simulink model "sim_all"  (R2020a)
settings: Solver=VariableStepAuto  StartTime=0.0  StopTime=2000  RelTol=1e-3
values from neighbouring files (symbols this model uses):
  a1 = rho * D^4 * alpha1    (= 0.000388302366464)    [data_current.m]
  a2 = -rho * D^3 * alpha2 * (1 - omega)    (= 0.0037030698432)    [data_current.m]
  alpha1 = 0.0113    [data_current.m]
  alpha2 = -0.0091    [data_current.m]
  cornerA = [43.781381 ... (first row only)    [missionC.m]
  cornerB = [43.780975 ... (first row only)    [missionC.m]
  cornerC = [43.780189 ... (first row only)    [missionC.m]
  cornerD = [43.780602 ... (first row only)    [missionC.m]
  ctrl_clockwise = false    [controller.m]
  ctrl_int_bound_or = 0.1    [controller.m]
  ctrl_int_bound_pos = 1    [controller.m]
  ctrl_k_or = 1    [controller.m]
  ctrl_k_pos = 1/3    (= 0.333333333333)    [controller.m]
  ctrl_Ki_vel = 100    [controller.m]
  ctrl_Kp_v_pos = 200    [controller.m]
  ctrl_Kp_vel = 200    [controller.m]
  ctrl_TAM = [  1     1           0           0               0       0;               0     0           1           1               0       0;               0     0           0           0               1       1;               0     0  -(ctrl_r+ctrl_dc)  ctrl_r+ctrl_dc    0       0;               0     0           0           0            -ctrl_r    ctrl_r;           -ctrl_r ctrl_r        0           0       ...(+19 chars)    [controller.m]
  ctrl_Ts = 0.1    [controller.m]
  ctrl_va_uncontrolled = 0.15    [controller.m]
  ctrl_vel_uncontrolled = 0.5    [controller.m]
  D = 0.076    [data_current.m]
  dead_zone_limit = 31.5    [data_current.m]
  depth = 5    [missionC.m]
  distanceFromWall = 8    [missionC.m]
  initInspectedSide = 2    [missionC.m]
  initPoint = [ 43.780796 ... (first row only)    [missionC.m]
  mod_A = pi*mod_R*mod_R    [model.m]
  mod_Cd_F = 0.45    [model.m]
  mod_Cd_M = 0.4    [model.m]
  mod_eta_init = [mod_xNorth; mod_yEast; -mod_zDown; 0; 0; 0]    [model.m]
  mod_g = 9.81    [model.m]
  mod_h0 = 0    [model.m]
  mod_Ixx = mod_Io(1,1)    [model.m]
  mod_Iyy = mod_Io(2,2)    [model.m]
  mod_Izz = mod_Io(3,3)    [model.m]
  mod_Kp_dot = 0    [model.m]
  mod_lat0 = 43.780189    [model.m]
  mod_lon0 = 11.282698    [model.m]
  mod_m = 100    [model.m]
  mod_Mq_dot = mod_Kp_dot    (= 0)    [model.m]
  mod_ni_init = [0; 0; 0; 0; 0; 0]    [model.m]
  mod_Nr_dot = mod_Kp_dot    (= 0)    [model.m]
  mod_p1 = [0; mod_R; 0]    [model.m]
  mod_p2 = [0; -mod_R; 0]    [model.m]
  mod_p3 = [0; 0; (mod_R + mod_z_cm)]    [model.m]
  mod_p4 = [0; 0; -(mod_R + mod_z_cm)]    [model.m]
  mod_p5 = [mod_R; 0; 0]    [model.m]
  mod_p6 = [-mod_R; 0; 0]    [model.m]
  mod_R = ((3*mod_Vol)/(4*pi))^(1/3)    [model.m]
  mod_Rm = (4*mod_R)/(3*pi)    [model.m]
  mod_t1 = [1; 0; 0]    [model.m]
  mod_t2 = [1; 0; 0]    [model.m]
  mod_t3 = [0; 1; 0]    [model.m]
  mod_t4 = [0; 1; 0]    [model.m]
  mod_t5 = [0; 0; 1]    [model.m]
  mod_t6 = [0; 0; 1]    [model.m]
  mod_W = mod_m*mod_g    (= 981)    [model.m]
  mod_Xu_dot = (2/3)*mod_rho_AUV*pi*(mod_R^3)    [model.m]
  mod_Yv_dot = mod_Xu_dot    [model.m]
  mod_z_cm = mod_r_cm(3)    [model.m]
  mod_Zw_dot = mod_Xu_dot    [model.m]
  n_max = 340    [data_current.m]
  nav_DT = 0.1    [navigation.m]
  nav_filter = -1    [data_analysis_simulation_total.m]    (also in navigation.m)
  nav_giro = 2    [navigation.m]
  nav_h0 = 0    [navigation.m]
  nav_lat0 = cornerC(1)    [navigation.m]
  nav_lon0 = cornerC(2)    [navigation.m]
  nav_plane_AB = coefficient_plane(nav_A,nav_B)    [navigation.m]
  nav_plane_BC = coefficient_plane(nav_B,nav_C)    [navigation.m]
  nav_plane_CD = coefficient_plane(nav_C,nav_D)    [navigation.m]
  nav_plane_DA = coefficient_plane(nav_D,nav_A)    [navigation.m]
  nav_resampling = 10000    [navigation.m]
  omega = 0.1    [data_current.m]
  relativeDirection = 30    [missionC.m]
  res_enable_n_eff = 1    [navigation.m]
  rho = 1030    [data_current.m]
  sens_distCM = 0.267    [sensors.m]
  sens_Sample_time_AHRS = 0.1    [sensors.m]
  sens_Sample_time_depth = 0.1    [sensors.m]
  sens_Sample_time_dvl = 0.2    [sensors.m]
  sens_Sample_time_GPS = 1    [sensors.m]
  sens_Sample_time_GYRO = 0.1    [sensors.m]
  sens_Sample_time_sonar = 0.5    [sensors.m]
  sens_threshold = 0.485    [sensors.m]
  sens_Variance_AHRS_pitch = (0.0087)^2    (= 7.569e-05)    [sensors.m]
  sens_Variance_AHRS_roll = (0.0087)^2    (= 7.569e-05)    [sensors.m]
  sens_Variance_AHRS_yaw = (0.0017)^2    (= 2.89e-06)    [sensors.m]
  sens_Variance_depth1 = (0.2)^2    (= 0.04)    [sensors.m]
  sens_Variance_depth2 = (0.4)^2    (= 0.16)    [sensors.m]
  sens_Variance_DVL = (speed*0.03)^2    [sensors.m]
  sens_Variance_GPS = 3    [sensors.m]
  sens_Variance_GYRO = 2.5133e-06    [sensors.m]
  sens_Variance_sonar = 0.05    [sensors.m]
  soglia_or = [0.1, 0.1, 0.1]    [mission.m]
  soglia_orp = 0.1    [mission.m]
  soglia_parete = 0.5    [mission.m]
  soglia_parete_frenata = 0.5    [mission.m]
  soglia_pos = [0.00001, 0.00001, 0.5]    [mission.m]
  soglia_SOS_collisione = 2    [mission.m]
  soglia_SOS_or = [0.25, 0.25, 0.25]    [mission.m]
  soglia_SOS_orp = 0.25    [mission.m]
  soglia_SOS_parete = 1    [mission.m]
  soglia_SOS_pos = [0.00005, 0.00005, 1]    [mission.m]
  soglia_SOS_pos_ris = 2    [mission.m]
  soglia_SOS_vel = 0.2    [mission.m]
  SOS = 0    [mission.m]
  speed = 0.4    [missionC.m]
  stato = 100    [mission.m]
  timer = 40*2    (= 80)    [mission.m]
  Ts_supervisor = 0.1    [mission.m]
undefined symbols (not defined in the file or in its folder): DiscIntNeverNeededParam, nav_A, nav_B, nav_C, nav_D
libraries: simulink x8, cstblocks x6, simulink_extras x1
(part 5 of 8)

== matlab function sim_all/EKF/Calcolo distaza pareti/Calcolo orientazione dalla parete ==
  data: pos_es input; orient_parete output; parete_attuale input; orient input; nav_plane_AB parameter; nav_plane_BC parameter; nav_plane_CD parameter; nav_plane_DA parameter
function orient_parete  = orient_parete_calculator(pos_es, parete_attuale, orient, nav_plane_AB, nav_plane_BC, nav_plane_CD, nav_plane_DA)
    
    %consideriamo angoli di pitch e roll nulli, cioè si calcola
    %l'orientazione rispetto alla parete solo considerando rotazioni di yaw
    %(piano xy)

    Yaw   = orient(3);
    R_z = [cos(Yaw)     sin(Yaw)       0     ;
           -sin(Yaw)    cos(Yaw)       0     ;
              0            0           1    ];
    v_pos= R_z'*[1 0 0]';  %versore della retta lungo l'asse x (in body) in NED,
                       %cioè la direzione di riferimento di prua del veicolo     
    
    %selezione della parete di pattugliamento
switch parete_attuale                      
    case 1
        %% Piano di pattugliamento AB
        versore_plane_NED = [nav_plane_AB(1) nav_plane_AB(2) 0]';    %versore normale al piano
        versore_plane_NED = versore_plane_NED/norm(versore_plane_NED);

        %calcolo distanza e intersezione lungo la normale al piano
        t_ = -(pos_es(1)+nav_plane_AB(2)*pos_es(2)+nav_plane_AB(4))/(nav_plane_AB(2)*versore_plane_NED(2)+versore_plane_NED(1));
        inter_perp=zeros(3,1);
        inter_perp(1) = pos_es(1) + versore_plane_NED(1)*t_;
        inter_perp(2) = pos_es(2) + versore_plane_NED(2)*t_;
        inter_perp(3) = pos_es(3) + versore_plane_NED(3)*t_;
        
        %calcolo distanza e intersezione lungo la direzione di prua
        t_ = -(pos_es(1)+nav_plane_AB(2)*pos_es(2)+nav_plane_AB(4))/(nav_plane_AB(2)*v_pos(2)+v_pos(1));
        inter_prua=zeros(3,1);
        inter_prua(1) = pos_es(1) + v_pos(1)*t_;
        inter_prua(2) = pos_es(2) + v_pos(2)*t_;
        inter_prua(3) = pos_es(3) + v_pos(3)*t_;
        
        coef = nav_plane_AB;
        coef(4)=[];
        orient_parete = rad2deg(asin(abs(coef*v_pos)/(norm(coef)*norm(v_pos))));
        %se orient_parete è positiva, allora ci si trova tra - 90 e + 90 rispetto alla normale della parete 
        if t_ > 0              
            if inter_prua(1) > inter_perp(1) && inter_prua(2) < inter_perp(2)
                orient_parete = orient_parete - 90;
            else
                orient_parete = -(orient_parete - 90);
            end
        else
            if inter_prua(1) > inter_perp(1) && inter_prua(2) < inter_perp(2)
                orient_parete = (orient_parete + 90);
            else
                orient_parete = -(orient_parete + 90);
            end
        end    
    case 2
        %% Piano di pattugliamento BC
      	versore_plane_NED = [nav_plane_BC(1) nav_plane_BC(2) 0]';    %versore normale al piano
        versore_plane_NED = versore_plane_NED/norm(versore_plane_NED);

        %calcolo distanza e intersezione lungo la normale al piano
        t_ = -(pos_es(1)+nav_plane_BC(2)*pos_es(2)+nav_plane_BC(4))/(nav_plane_BC(2)*versore_plane_NED(2)+versore_plane_NED(1));
        inter_perp=zeros(3,1);
        inter_perp(1) = pos_es(1) + versore_plane_NED(1)*t_;
        inter_perp(2) = pos_es(2) + versore_plane_NED(2)*t_;
        inter_perp(3) = pos_es(3) + versore_plane_NED(3)*t_;

        %calcolo distanza e intersezione lungo la direzione di prua
        t_ = -(pos_es(1)+nav_plane_BC(2)*pos_es(2)+nav_plane_BC(4))/(nav_plane_BC(2)*v_pos(2)+v_pos(1));
        inter_prua=zeros(3,1);
        inter_prua(1) = pos_es(1) + v_pos(1)*t_;
        inter_prua(2) = pos_es(2) + v_pos(2)*t_;
        inter_prua(3) = pos_es(3) + v_pos(3)*t_;
        
        coef = nav_plane_BC;
        coef(4)=[];
        v_pos=-v_pos;
        orient_parete = rad2deg(asin(abs(coef*v_pos)/(norm(coef)*norm(v_pos))));
        %se orient_parete è positiva, allora ci si trova tra - 90 e + 90 rispetto alla normale della parete 
        if t_ > 0              
            if inter_prua(1) > inter_perp(1) && inter_prua(2) > inter_perp(2)
                orient_parete = orient_parete - 90;
            else
                orient_parete = -(orient_parete - 90);
            end
        else
            if inter_prua(1) > inter_perp(1) && inter_prua(2) > inter_perp(2)
                orient_parete = orient_parete + 90;
            else
                orient_parete = -(orient_parete + 90);
            end
        end
        
    case 3
        %% Piano di pattugliamento CD
      	versore_plane_NED = [nav_plane_CD(1) nav_plane_CD(2) 0]';    %versore normale al piano
        versore_plane_NED = versore_plane_NED/norm(versore_plane_NED);

        %calcolo distanza e intersezione lungo la normale al piano
        t_ = -(pos_es(1)+nav_plane_CD(2)*pos_es(2)+nav_plane_CD(4))/(nav_plane_CD(2)*versore_plane_NED(2)+versore_plane_NED(1));
        inter_perp=zeros(3,1);
        inter_perp(1) = pos_es(1) + versore_plane_NED(1)*t_;
        inter_perp(2) = pos_es(2) + versore_plane_NED(2)*t_;
        inter_perp(3) = pos_es(3) + versore_plane_NED(3)*t_;

        %calcolo distanza e intersezione lungo la direzione di prua
        t_ = -(pos_es(1)+nav_plane_CD(2)*pos_es(2)+nav_plane_CD(4))/(nav_plane_CD(2)*v_pos(2)+v_pos(1));
        inter_prua=zeros(3,1);
        inter_prua(1) = pos_es(1) + v_pos(1)*t_;
        inter_prua(2) = pos_es(2) + v_pos(2)*t_;
        inter_prua(3) = pos_es(3) + v_pos(3)*t_;
        
        coef = nav_plane_CD;
        coef(4)=[];
        v_pos=-v_pos;
        orient_parete = rad2deg(asin(abs(coef*v_pos)/(norm(coef)*norm(v_pos))));
        %se orient_parete è positiva, allora ci si trova tra - 90 e + 90 rispetto alla normale della parete 
        if t_ > 0              
            if inter_prua(1) > inter_perp(1) && inter_prua(2) < inter_perp(2)
                orient_parete = -orient_parete + 90;
            else
                orient_parete = orient_parete - 90;
            end
        else
             if inter_prua(1) > inter_perp(1) && inter_prua(2) < inter_perp(2)
                orient_parete = -orient_parete - 90;
            else
                orient_parete = orient_parete + 90;
            end
        end
        
    case 4
        %% Piano di pattugliamento DA
      	versore_plane_NED = [nav_plane_DA(1) nav_plane_DA(2) 0]';    %versore normale al piano
        versore_plane_NED = versore_plane_NED/norm(versore_plane_NED);

        %calcolo distanza e intersezione lungo la normale al piano
        t_ = -(pos_es(1)+nav_plane_DA(2)*pos_es(2)+nav_plane_DA(4))/(nav_plane_DA(2)*versore_plane_NED(2)+versore_plane_NED(1));
        inter_perp=zeros(3,1);
        inter_perp(1) = pos_es(1) + versore_plane_NED(1)*t_;
        inter_perp(2) = pos_es(2) + versore_plane_NED(2)*t_;
        inter_perp(3) = pos_es(3) + versore_plane_NED(3)*t_;

        %calcolo distanza e intersezione lungo la direzione di prua
        t_ = -(pos_es(1)+nav_plane_DA(2)*pos_es(2)+nav_plane_DA(4))/(nav_plane_DA(2)*v_pos(2)+v_pos(1));
        inter_prua=zeros(3,1);
        inter_prua(1) = pos_es(1) + v_pos(1)*t_;
        inter_prua(2) = pos_es(2) + v_pos(2)*t_;
        inter_prua(3) = pos_es(3) + v_pos(3)*t_;
        
        coef = nav_plane_DA;
        coef(4)=[];
        orient_parete = rad2deg(asin(abs(coef*v_pos)/(norm(coef)*norm(v_pos))));
        %se orient_parete è positiva, allora ci si trova tra - 90 e + 90 rispetto alla normale della parete 
        if t_ > 0              
            if inter_prua(1) < inter_perp(1) && inter_prua(2) < inter_perp(2)
                orient_parete = orient_parete - 90;
            else
                orient_parete = -orient_parete + 90;
            end
        else
            if inter_prua(1) < inter_perp(1) && inter_prua(2) < inter_perp(2)
                orient_parete = orient_parete + 90;
            else
                orient_parete = -orient_parete - 90;
            end
        end
        
    otherwise
        %%
       coef=[0 0 0 0];
       orient_parete = NaN;
end
    
    
end

== matlab function sim_all/EKF/ECEF2NED ==
  data: GPS_ECEF input; GPS_NED output; nav_lat0 parameter; nav_lon0 parameter; nav_h0 parameter
%Componente di ingresso in terna ECEF
%Lat  [gradi]
%Long  [gradi]
%flag data_valid

function GPS_NED = GPS_conv_valid(GPS_ECEF, nav_lat0, nav_lon0, nav_h0)
    
    coder.extrinsic('evalin', 'wgs84Ellipsoid', 'geodetic2ned');

    if GPS_ECEF(3)==1
        GPS_NED = zeros(3,1);
        [GPS_NED(1),GPS_NED(2),GPS_NED(3)]= geodetic2ned(GPS_ECEF(1),GPS_ECEF(2),0,nav_lat0,nav_lon0,nav_h0,wgs84Ellipsoid);
        GPS_NED(3) = GPS_ECEF(3);
    else                            %qui non si effettua la conversione se il dato non è valido
        GPS_NED = GPS_ECEF; 
    end
end

== matlab function sim_all/EKF/Extended Kalman Filter/AHRS__check/MATLAB Function4 ==
  data: flag_AHRS output; AHRS_new input; AHRS_now output; AHRS_old input
%gestione di misura errata di AHRS
function [flag_AHRS, AHRS_now] = fcn(AHRS_new, AHRS_old)

    if isnan(AHRS_new(1,1)) || isnan(AHRS_new(2,1)) || isnan(AHRS_new(3,1))
        AHRS_now = AHRS_old;
        flag_AHRS = 1;
        disp('Misura AHRS non valida')
    else
        AHRS_now = AHRS_new;
        flag_AHRS = 0;
    end  
end

== matlab function sim_all/EKF/Extended Kalman Filter/CORREZIONE/MATLAB Function ==
  data: x_k_k_1 input; x_k output; P_k_k_1 input; e input size=6 1; H input size=6 3; R_k input size=6 6; P_k output; nav_flag_init input
%%Passo di Correzione

function [x_k, P_k] = correction(x_k_k_1,P_k_k_1, e, H, R_k,nav_flag_init)
    
     x_k = zeros(3,1);
     P_k = zeros(3,3);
     
     
    if nav_flag_init ~= 0
        %matrice ottenuta da derivata di funzione h (6x1) per i rumori sei vari
        %sensori, che sono 6. (ha dimensione 6x6)
        %andrebbero anche considerati i rumori legati all'AHRS che al momento
        %sono trascurati
        %M = eye(6,6);              %M è l'dientità
        S_k = H*P_k_k_1*H'+ R_k;
        K_k = P_k_k_1*H'*(inv(S_k));

        P_k = (eye(3)-(K_k*H))*P_k_k_1;
        x_k = x_k_k_1 + K_k * e;
    end

end

== matlab function sim_all/Mission_supervisor_v3/Mission_Supervisor/Immersione/MATLAB Function ==
  data: soglia_pos parameter; delta_current_immers output; delta_stato_immers output; Pos_d output size=3; Or_d output size=3; Pos_s input; depth parameter; punto_iniz_patt input; Or_in input; error_flag input; soglia_SOS_pos parameter; SOS parameter
function [delta_current_immers, delta_stato_immers, Pos_d, Or_d]=Immersione(soglia_pos, Pos_s, depth, punto_iniz_patt, Or_in, error_flag, soglia_SOS_pos, SOS)

    disp("Immersione");
    
    %% Unità di misura 
    
    % Pos_d, Pos_s, punto_iniz_patt, soglia_pos, soglia_SOS_pos            [deg, deg, m]
    % Or_d, Or_in                                                          [rad, rad, rad]
    % distanceFromWall, depth                                              [m]


    %% Inizializzazione variabili
    
    % Utilizzata durante la permanenza nello stato corrente
    delta_stato_immers = 0;
    
    pronti = false; 
    
    %% Preparazione dei riferimenti da fornire ai blocchi successivi
    
    % Posizione da raggiungere
    Pos_d = [punto_iniz_patt(1); punto_iniz_patt(2); depth];
                                                                            %*****TEST******%
                                                                            %Pos_d = [43; 11; 0];
    
    % Orientazione da mantenere
    Or_d = Or_in;
    
    % Transizione di stato effettiva
    delta_current_immers = 103 - 102;  
        
       
    %% Verifiche
    
    % Verifica della corretta posizione
    if (abs(Pos_s(1) - Pos_d(1)) > soglia_SOS_pos(1) || ...
        abs(Pos_s(2) - Pos_d(2)) > soglia_SOS_pos(2))
    
        SOS = 1;
        disp("EMERGENZA:"); 
        
        if (abs(Pos_s(1) - Pos_d(1)) > soglia_SOS_pos(1))
            disp("Rilevato errore sulla posizione X");
        end
        
        if (abs(Pos_s(2) - Pos_d(2)) > soglia_SOS_pos(2))
            disp("Rilevato errore sulla posizione Y");
        end

    end
    
    if error_flag == 1
        disp("EMERGENZA: errore segnalato dagli altri sottosistemi");
        SOS = 1;
    end
    
    % Si verifica di aver raggiunto la profondità desiderata 
    if (SOS == 0 && ...
        abs(Pos_s(3) - Pos_d(3)) < soglia_pos(3))
    
        pronti = true;
    end
    
    
    %% Decisione dello stato successivo
    
    if pronti == true
        
        delta_stato_immers = 104 - 103; % Transizione eseguita correttamente
    end 
    if SOS == 1
            
            delta_stato_immers = 301 - 103; % Transizione nello stato di emergenza
    end
    % Si rimane nello stato corrente

end

== matlab function sim_all/EKF/Extended Kalman Filter/Creazione vettore delle misure ==
  data: flag_vect output; GPS input; mis_vect output; depth input; s_pr input; s_dx input; s_sx input; mis_vect_prec input; J input; pos input; nav_plane_AB parameter; nav_plane_BC parameter; nav_plane_CD parameter; nav_plane_DA parameter; nav_A parameter; nav_B parameter; nav_C parameter; nav_D parameter; distanceFromWall parameter; flag_DVL input; flag_AHRS input
%%
% Questa funzione impila le informazioni derivanti dai vari sensori in un
% unico vettore mis_vect 7x1.                                 
% Ci sarà un corrispondente vettore flag_vect 7x1 di flag che sarà pari a:

% flag(i) = 0  se la misura è uguale a quella arrivata nell'istante
% predecente, in tal caso la correzione non verrà effettuata
% flag(i) = 1 se la misura è stata aggiornata rispetto a quella precendente
 
% NB il controllo sulla validità dei dati del GPS è valutata nel blocco
% sucessivo

function [flag_vect,mis_vect] = misure_vector(GPS,depth,s_pr,s_dx,s_sx, mis_vect_prec,...
          J, pos, nav_plane_AB, nav_plane_BC, nav_plane_CD, nav_plane_DA, nav_A, nav_B, nav_C, nav_D, distanceFromWall, ...
          flag_DVL, flag_AHRS)
    
    mis_vect = zeros(7,1);
    flag_vect = zeros(7,1);
	mis_vect = [GPS(1) GPS(2) GPS(3) depth s_pr s_dx s_sx]';
    
    for i=[1:7]
        if mis_vect(i) ~= mis_vect_prec(i)
            flag_vect(i) = 1;
        end
    end
    
    %si valuta se la misura del profondimetro è valida
    if isnan(depth)  
        flag_vect(4) = 0;
    end
     
    %si controlla che sia disponibile il dato dai sonar
    if isnan(s_pr)
        flag_vect(5) = 0;
    end
    if isnan(s_dx)
        flag_vect(6) = 0;
    end
    if isnan(s_sx)
        flag_vect(7) = 0;
    end
    
    %se i dati dei sonar qui sono utilizzabili, è necessario assicurarci che il 
    %loro raggio non punti verso uno spigolo, in quel caso potrebbe
    %causare una correzione errata
    if flag_vect(5) == 1               %se i dati del sonar di prua sono nuovi
            versore_son_NED = J*[1 0 0]';          %versore terna NED sonar prua
            flag_vect(5) = inter(pos, versore_son_NED ,nav_plane_AB,nav_plane_BC,nav_plane_CD,nav_plane_DA, nav_A, nav_B, nav_C, nav_D);       
    end

        if flag_vect(6) == 1               %se i dati del sonar destro sono nuovi
                versore_son_NED = J*[0 1 0]';          %versore terna NED sonar dx
                flag_vect(6) = inter(pos, versore_son_NED ,nav_plane_AB,nav_plane_BC,nav_plane_CD,nav_plane_DA, nav_A, nav_B, nav_C, nav_D);       
        end
        if flag_vect(7) == 1               %se i dati del sonar sinistro sono nuovi
                versore_son_NED = J*[0 -1 0]';          %versore terna NED sonar sx
                flag_vect(7) = inter(pos, versore_son_NED ,nav_plane_AB,nav_plane_BC,nav_plane_CD,nav_plane_DA, nav_A, nav_B, nav_C, nav_D);
        end 
%         la terza componente di flag_vect non sarà utilizzata. per assicurarci
%         che i dati del GPS siano validi ci rifaremo sempre su mis_vect


    if flag_DVL == 0 && flag_AHRS == 0  %i sonar vengono usati sempre nella correzione se un sensore tra DLV
                                        %o AHRS non funziona momentaneamente 
        
        soglia_distanza=distanceFromWall*3;
        soglia_variazione=0.8;
        if  mis_vect(5) > soglia_distanza || abs(mis_vect(5)- mis_vect_prec(5)) > soglia_variazione
            flag_vect(5) = 0;
        end
        if  mis_vect(6) > soglia_distanza || abs(mis_vect(6)- mis_vect_prec(6)) > soglia_variazione
            flag_vect(6) = 0;
        end
        if  mis_vect(7) > soglia_distanza || abs(mis_vect(7)- mis_vect_prec(7)) > soglia_variazione
            flag_vect(7) = 0;
        end
    end
end




function [flag] = inter(pos, versore_son_NED,nav_plane_AB,nav_plane_BC,nav_plane_CD,nav_plane_DA, nav_A, nav_B, nav_C, nav_D)
    
    %calcolo della distanza dalla posizione ai piani delle pareti seguendo
    %la direzione data dal versore del sonar

    t_AB = -(pos(1)+nav_plane_AB(2)*pos(2)+nav_plane_AB(4))/(nav_plane_AB(2)*versore_son_NED(2)+versore_son_NED(1));
    t_BC = -(pos(1)+nav_plane_BC(2)*pos(2)+nav_plane_BC(4))/(nav_plane_BC(2)*versore_son_NED(2)+versore_son_NED(1));
    t_CD = -(pos(1)+nav_plane_CD(2)*pos(2)+nav_plane_CD(4))/(nav_plane_CD(2)*versore_son_NED(2)+versore_son_NED(1));
    t_DA = -(pos(1)+nav_plane_DA(2)*pos(2)+nav_plane_DA(4))/(nav_plane_DA(2)*versore_son_NED(2)+versore_son_NED(1));
    
    if t_AB < 0
        t_AB = inf;
    end
    if t_BC < 0
        t_BC = inf;
    end
    if t_CD < 0
        t_CD = inf;
    end
    if t_DA < 0
        t_DA = inf;
    end
           
    [dist, index] = min([t_AB t_BC t_CD t_DA]);
    dist = dist - 0.267;       %va tolto il raggio del veicolo rispetto al centro di massa
    
    int=zeros(1,3);
    %calcolo l'intersezione
    int(1) = pos(1) + versore_son_NED(1)*dist;
    int(2) = pos(2) + versore_son_NED(2)*dist;
    int(3) = 0;
    
    soglia_spigolo = 5;          %distanza massima dallo spigolo entro la quale 
                       %la misura del sonar non è buona
    flag=1;
    switch index
        case 1      
            if norm(int-nav_A) < soglia_spigolo || norm(int-nav_B) < soglia_spigolo
                flag=0;
            end
        case 2
            if norm(int-nav_B) < soglia_spigolo || norm(int-nav_C) < soglia_spigolo
                flag=0;
            end
        case 3
            if norm(int-nav_C) < soglia_spigolo || norm(int-nav_D) < soglia_spigolo
                flag=0;
            end
        case 4
            if norm(int-nav_D) < soglia_spigolo || norm(int-nav_A) < soglia_spigolo
                flag=0;
            end
        otherwise
            disp('errore nella intersezione del piano')
    end
end

== matlab function sim_all/EKF/Extended Kalman Filter/DVL_check/MATLAB Function4 ==
  data: flag_DVL output; DVL_new input; DVL_now output; DVL_old input
%gestione di misura errata del DVL
function [flag_DVL, DVL_now] = fcn(DVL_new, DVL_old)

    if isnan(DVL_new(1,1)) || isnan(DVL_new(2,1)) || isnan(DVL_new(3,1))
        DVL_now = DVL_old;
        flag_DVL = 1;
        disp('Misura DVL non valida')
    else
        DVL_now = DVL_new;
        flag_DVL = 0;
    end  
end

== matlab function sim_all/EKF/Extended Kalman Filter/MATLAB Function ==
  data: GPS input; x0 output; depth input; P0 output; flag input; flag output
%blocco di inizializzazione del Filtro

function [x0, P0, flag] = EKF_init(GPS, depth, flag)
    
    x0 = zeros(3,1);
    P0 = zeros(3,3);
    
    % il valore di nav_flag_init è all'inizio della simulazione pari a 0
    % appena c'è il primo dato disponibile del GPS (insieme al profondimetro)
    % si assume quella come punto di inizializzazione del filtro.

    if flag == 0
        if GPS(3)==1
            x0 = [GPS(1), GPS(2), depth]';
            P0 = diag([3 3 (0.2)^2]);       %sono le varianze del GPS e del profondimetro (come nella R)
            flag = 1;                   %se vale 1 bisogna assegnare i primi valori a x_k_1 e P_k_1
        end
               
    end

end

== matlab function sim_all/EKF/Extended Kalman Filter/MATLAB Function1 ==
  data: orient input; J output
%calcolo matrice J
function J = calcolo_jacobiano(orient)

    Roll  = orient(1);
    Pitch = orient(2);
    Yaw   = orient(3);

    R_x = [ 1               0              0;
            0           cos(Roll)     sin(Roll);
            0           -sin(Roll)    cos(Roll)];

    R_y = [cos(Pitch)       0   -sin(Pitch);
              0             1         0;
           sin(Pitch)       0   cos(Pitch)];

    R_z = [cos(Yaw)     sin(Yaw)      0;
          -sin(Yaw)     cos(Yaw)      0;
              0            0          1];

    J = (R_z'*R_y')*R_x';
end

== matlab function sim_all/EKF/Extended Kalman Filter/MATLAB Function2 ==
  data: u_k_1 input; orient input; L output
%calcolo matrice L
function L = calcolo_L(u_k_1,orient)

    L =  [   u_k_1(2)*((sin(orient(1))*sin(orient(3)))/10 + (cos(orient(1))*cos(orient(3))*sin(orient(2)))/10) + u_k_1(3)*((cos(orient(1))*sin(orient(3)))/10 - (cos(orient(3))*sin(orient(1))*sin(orient(2)))/10), (u_k_1(3)*cos(orient(1))*cos(orient(3))*cos(orient(2)))/10 - (u_k_1(1)*cos(orient(3))*sin(orient(2)))/10 + (u_k_1(2)*cos(orient(3))*cos(orient(2))*sin(orient(1)))/10, u_k_1(3)*((cos(orient(3))*sin(orient(1)))/10 - (cos(orient(1))*sin(orient(3))*sin(orient(2)))/10) - u_k_1(2)*((cos(orient(1))*cos(orient(3)))/10 + (sin(orient(1))*sin(orient(3))*sin(orient(2)))/10) - (u_k_1(1)*cos(orient(2))*sin(orient(3)))/10, (cos(orient(3))*cos(orient(2)))/10, (cos(orient(3))*sin(orient(1))*sin(orient(2)))/10 - (cos(orient(1))*sin(orient(3)))/10, (sin(orient(1))*sin(orient(3)))/10 + (cos(orient(1))*cos(orient(3))*sin(orient(2)))/10;...
           - u_k_1(2)*((cos(orient(3))*sin(orient(1)))/10 - (cos(orient(1))*sin(orient(3))*sin(orient(2)))/10) - u_k_1(3)*((cos(orient(1))*cos(orient(3)))/10 + (sin(orient(1))*sin(orient(3))*sin(orient(2)))/10), (u_k_1(3)*cos(orient(1))*cos(orient(2))*sin(orient(3)))/10 - (u_k_1(1)*sin(orient(3))*sin(orient(2)))/10 + (u_k_1(2)*cos(orient(2))*sin(orient(1))*sin(orient(3)))/10, u_k_1(3)*((sin(orient(1))*sin(orient(3)))/10 + (cos(orient(1))*cos(orient(3))*sin(orient(2)))/10) - u_k_1(2)*((cos(orient(1))*sin(orient(3)))/10 - (cos(orient(3))*sin(orient(1))*sin(orient(2)))/10) + (u_k_1(1)*cos(orient(3))*cos(orient(2)))/10, (cos(orient(2))*sin(orient(3)))/10, (cos(orient(1))*cos(orient(3)))/10 + (sin(orient(1))*sin(orient(3))*sin(orient(2)))/10, (cos(orient(1))*sin(orient(3))*sin(orient(2)))/10 - (cos(orient(3))*sin(orient(1)))/10;...
                                                                                                             (u_k_1(2)*cos(orient(1))*cos(orient(2)))/10 - (u_k_1(3)*cos(orient(2))*sin(orient(1)))/10,                                      - (u_k_1(1)*cos(orient(2)))/10 - (u_k_1(3)*cos(orient(1))*sin(orient(2)))/10 - (u_k_1(2)*sin(orient(1))*sin(orient(2)))/10,                                                                                                                                                                                                                              0,               -sin(orient(2))/10,                                               (cos(orient(2))*sin(orient(1)))/10,                                               (cos(orient(1))*cos(orient(2)))/10]; 
end

== matlab function sim_all/EKF/Extended Kalman Filter/MATLAB Function3 ==
  data: flag_vect input; mis_vect input; R_ input size=6 6; R_k output size=6 6
%calcolo matrice R
function R_k = R_cutter(flag_vect, mis_vect,R_)
%valutazione misure GPS
    R=R_;   
    i=0;
    if mis_vect(3) == 0                    %se i dati del GPS non sono validi
        R(1,:) = [];
        R(:,1) = [];
        i=i+1;
        R(2-i,:) = [];
        R(:,2-i) = [];
        i=i+1;
        if flag_vect(4) == 0               %se i dati del profondimetro non sono nuovi
            R(3-i,:) = [];
            R(:,3-i) = [];
            i=i+1;
        end
        if flag_vect(5) == 0               %se i dati del sonar di prua non sono nuovi
            R(4-i,:) = [];
             R(:,4-i) = [];
            i=i+1;
        end
        if flag_vect(6) == 0               %se i dati del sonar sinistro non sono nuovi
            R(5-i,:) = [];
             R(:,5-i) = [];
            i=i+1;
        end
        if flag_vect(7) == 0               %se i dati del sonar destro non sono nuovi
            R(6-i,:) = [];
             R(:,6-i) = [];
        end
    % da qui invece abbiamo il GPS valido
    else
        if flag_vect(1)==0 || flag_vect(2)==0  %se i dati del GPS non sono nuovi
            R(1-i,:) = [];
            R(:,1-i) = [];
            i=i+1;
            R(2-i,:) = [];
            R(:,2-i) = [];
            i=i+1;
        end
       
        if flag_vect(4) == 0               %se i dati del profondimetro non sono nuovi
            R(3-i,:) = [];
            R(:,3-i) = [];
            i=i+1;
        end
       
        R(4-i,:) = []; %annulliamo le misure dei sonar
        R(:,4-i) = [];         
        i=i+1;
        R(5-i,:) = [];
        R(:,5-i) = [];
        i=i+1;
        R(6-i,:) = [];
        R(:,6-i) = [];
       
    end
    R_k=R;
end

== matlab function sim_all/EKF/Extended Kalman Filter/MISURA VIRTUALE/MATLAB Function ==
  data: x_k_k_1 input; flag_vect input; mis_vect input; e output size=6 1; H output size=6 3; J input; nav_plane_AB parameter; nav_plane_BC parameter; nav_plane_CD parameter; nav_plane_DA parameter
%calcolo  misure virtuali
function [e, H] = virtual(x_k_k_1, flag_vect, mis_vect, J, nav_plane_AB, nav_plane_BC, nav_plane_CD, nav_plane_DA)

    e = zeros(6,1);
    h = zeros(6,1);
    z = zeros(6,1);
    H = zeros(6,3);
    
    
    %valutazione misure GPS
    if mis_vect(3)==1                                   %se i dati del GPS sono validi
        if flag_vect(1) == 1 && flag_vect(2) == 1       %se i dati del GPS sono nuovi
            
            z = z + [mis_vect(1) mis_vect(2) 0 0 0 0]';
            h = h + [x_k_k_1(1)   x_k_k_1(2) 0 0 0 0]';
        
            H(1,:)= [1 0 0];
            H(2,:)= [0 1 0];
        end
    end
    
    %valutazione misure depth
    if flag_vect(4) == 1                                 %se i dati del profondimetro sono nuovi
            
        z = z + [0 0 mis_vect(4) 0 0 0]'; 
        h = h + [0 0  x_k_k_1(3) 0 0 0]';

        H(3,:)= [0 0 1];
    end
    
    %valutiamo ora le misure virtuali solo se quelle del GPS non sono
    %valide
    if mis_vect(3)==0                      %se i dati del GPS non sono validi
        
        if flag_vect(5) == 1               %se i dati del sonar di prua sono nuovi
                
                versore_son_NED = J*[1 0 0]';          %versore terna NED sonar prua
                
                [distanza, plane] = inter(x_k_k_1, versore_son_NED ,nav_plane_AB,nav_plane_BC,nav_plane_CD,nav_plane_DA);
                z = z + [0 0 0 mis_vect(5) 0 0]'; 
                h = h + [0 0 0 distanza    0 0]';
                
                H_new=zeros(1,3);
                [H_new(1), H_new(2), H_new(3)] = calc_H_vect(x_k_k_1, versore_son_NED,plane);
                H(4,:) = H_new;                
        end
    
        if flag_vect(6) == 1               %se i dati del sonar destro sono nuovi
                
                versore_son_NED = J*[0 1 0]';          %versore terna NED sonar dx
                
                [distanza, plane] = inter(x_k_k_1, versore_son_NED ,nav_plane_AB,nav_plane_BC,nav_plane_CD,nav_plane_DA);
                z = z + [0 0 0 0 mis_vect(6) 0]'; 
                h = h + [0 0 0 0 distanza    0]';
                
                H_new=zeros(1,3);
                [H_new(1), H_new(2), H_new(3)] = calc_H_vect(x_k_k_1, versore_son_NED,plane);
                H(5,:) = H_new;
        end
    
        if flag_vect(7) == 1               %se i dati del sonar sinistro sono nuovi
                 
                versore_son_NED = J*[0 -1 0]';          %versore terna NED sonar sx
                
                [distanza, plane] = inter(x_k_k_1, versore_son_NED ,nav_plane_AB,nav_plane_BC,nav_plane_CD,nav_plane_DA);
                z = z + [0 0 0 0 0 mis_vect(7)]'; 
                h = h + [0 0 0 0 0 distanza   ]'; 
                
                H_new=zeros(1,3);
                [H_new(1), H_new(2), H_new(3)] = calc_H_vect(x_k_k_1, versore_son_NED,plane);
                H(6,:) = H_new;
        end
    end
    
    e = z - h;
    
    %%si riducono le dimensioni della matrice H e del vettore e
    
    i=0;
    if mis_vect(3) == 0                    %se i dati del GPS non sono validi
        H(1-i,:) = [];
        e(1-i) = [];
        i=i+1;
        H(2-i,:) = [];
        e(2-i) = [];
        i=i+1;
        if flag_vect(4) == 0               %se i dati del profondimetro non sono nuovi
            H(3-i,:) = [];
            e(3-i) = [];
            i=i+1;
        end
        if flag_vect(5) == 0               %se i dati del sonar di prua non sono nuovi
            H(4-i,:) = [];
            e(4-i) = [];
            i=i+1;
        end
        if flag_vect(6) == 0               %se i dati del sonar sinistro non sono nuovi
            H(5-i,:) = [];
            e(5-i) = [];
            i=i+1;
        end
        if flag_vect(7) == 0               %se i dati del sonar destro non sono nuovi
            H(6-i,:) = [];
            e(6-i) = [];
        end
    % da qui invece si ha il GPS valido
    else
        if flag_vect(1)==0 || flag_vect(2)==0  %se i dati del GPS non sono nuovi
            H(1-i,:) = [];
            e(1-i) = [];
            i=i+1;
            H(2-i,:) = [];
            e(2-i) = [];
            i=i+1;
        end
        
        if flag_vect(4) == 0               %se i dati del profondimetro non sono nuovi
            H(3-i,:) = [];
            e(3-i) = [];
            i=i+1;
        end
        
        H(4-i,:) = [];                      %annulliamo le misure dei sonar
        e(4-i) = [];
        i=i+1;
        H(5-i,:) = [];
        e(5-i) = [];
        i=i+1;
        H(6-i,:) = [];        
        e(6-i) = [];    
    end
    i=0;
end



%%
%%%%%%%%%%%%%%%%%%%%%%%%%%%%%%%%%%%%%%%%%%%%%%%%%%%%%%%%%%%%%%%%%%%%%%%%%%%%%%%%%%%%%%%%

function [dist, plane] = inter(pos, versore_son_NED,nav_plane_AB,nav_plane_BC,nav_plane_CD,nav_plane_DA)
    
    %calcolo della distanza dalla posizione ai piani delle pareti seguendo
    %la direzione data dal versore del sonar

    t_AB = -(pos(1)+nav_plane_AB(2)*pos(2)+nav_plane_AB(4))/(nav_plane_AB(2)*versore_son_NED(2)+versore_son_NED(1));
    t_BC = -(pos(1)+nav_plane_BC(2)*pos(2)+nav_plane_BC(4))/(nav_plane_BC(2)*versore_son_NED(2)+versore_son_NED(1));
    t_CD = -(pos(1)+nav_plane_CD(2)*pos(2)+nav_plane_CD(4))/(nav_plane_CD(2)*versore_son_NED(2)+versore_son_NED(1));
    t_DA = -(pos(1)+nav_plane_DA(2)*pos(2)+nav_plane_DA(4))/(nav_plane_DA(2)*versore_son_NED(2)+versore_son_NED(1));
    
    if t_AB < 0
        t_AB = inf;
    end
    if t_BC < 0
        t_BC = inf;
    end
    if t_CD < 0
        t_CD = inf;
    end
    if t_DA < 0
        t_DA = inf;
    end
           
    [dist, index] = min([t_AB t_BC t_CD t_DA]);
    dist = dist - 0.267;       %va tolto il raggio del robot rispetto al centro di massa
    
    switch index
        case 1
            plane = nav_plane_AB;
        case 2
            plane = nav_plane_BC;
        case 3
            plane = nav_plane_CD;
        case 4
            plane = nav_plane_DA;
        otherwise
            plane=[0 0 0 0];
            disp('errore nella intersezione del piano')
    end
    
end

function [H1, H2, H3]= calc_H_vect(pos, sonar, plane)

    H1 = sign(pos(1) + plane(4) + pos(2)*plane(2))/abs(sonar(1) + plane(2)*sonar(2));
    H2 = (plane(2)*sign(pos(1) + plane(4) + pos(2)*plane(2)))/abs(sonar(1) + plane(2)*sonar(2));   
    H3 = 0;
end

== matlab function sim_all/EKF/Extended Kalman Filter/PREDIZIONE/Passo di Predizione ==
  data: x0 input; P0 input; x_k_1 input; u_k_1 input; x_k output; P_k_1 input; P_k output size=3 3; J input; L input; Q_k_1 input; nav_DT parameter; nav_flag_init input; nav_flag_init output
%% Passo di PREDIZIONE

function [x_k,  P_k, nav_flag_init] = prediction(x0, P0, x_k_1, u_k_1,  P_k_1, J, L, Q_k_1, nav_DT, nav_flag_init)
    
    x_k = zeros(3,1);
    P_k = zeros(3,3);

    % il valore di nav_flag_init all'inizio della simulazione é pari a 0
    % appena c'è il primo dato disponibile del GPS (insieme al profondimetro)
    % si assume quella come punto di inizializzazione del filtro.

    if nav_flag_init ~= 0      
        if nav_flag_init == 1
            x_k_1 = x0;
            P_k_1 = P0;
            nav_flag_init = 2;      % =2 così l'inizializzazione è fatta una sola volta.
        end
        
        %passo di predizione       
        x_k = x_k_1 + nav_DT*J*u_k_1;
        P_k = P_k_1 + L*Q_k_1*L';               %la matrice F è F = I
           
    end
end

== matlab function sim_all/EKF/Extended Kalman Filter/Q_error/MATLAB Function4 ==
  data: Q input; Q_k_1 input; Q_k output; flag_AHRS input; flag_DVL input
%calcolo matrice Q
function Q_k = fcn(Q, Q_k_1, flag_AHRS, flag_DVL)

    Q_k = Q;
    
    K=10;
    if flag_DVL == 1
       Q_k = Q_k_1 + K*5*diag([0,0,0,(0.012)^2,(0.012)^2,(0.012)^2]);
    end
    
    if flag_AHRS == 1
       Q_k = Q_k_1 + K*50*diag([(0.0087)^2, (0.0087)^2, (0.0017)^2,0,0,0]);  
    end
        
end

== matlab function sim_all/EKF/Gyro_check/MATLAB Function4 ==
  data: flag_gyro output; gyro_new input; gyro_now output; gyro_old input
% gestione di misura errata del giroscopio
function [flag_gyro, gyro_now] = fcn(gyro_new, gyro_old)

    if isnan(gyro_new(1,1)) || isnan(gyro_new(2,1)) || isnan(gyro_new(3,1))
        gyro_now = gyro_old;
        flag_gyro = 1;
        disp('Misura gyro non valida')
    else
        gyro_now = gyro_new;
        flag_gyro = 0;
    end  
end

== matlab function sim_all/EKF/MATLAB Function ==
  data: u input; y output
function y = Wrap2pi(u)
y = [0;0;0];
coder.extrinsic('wrapToPi');
y = wrapToPi(u);
end

== matlab function sim_all/EKF/NED2ECEF ==
  data: pos_es_NED input; pos_es_ECEF output; nav_lat0 parameter; nav_lon0 parameter; nav_h0 parameter
%%Blocco di conversione NED2ECEF

function pos_es_ECEF = pos_NED2ECEF(pos_es_NED,nav_lat0, nav_lon0, nav_h0)
     
    coder.extrinsic('evalin', 'wgs84Ellipsoid', 'ned2geodetic');
    pos_es_ECEF = zeros(3,1);
    depth = pos_es_NED(3); 
    
    [pos_es_ECEF(1),pos_es_ECEF(2),pos_es_ECEF(3)]= ned2geodetic(pos_es_NED(1),pos_es_NED(2),0,nav_lat0,nav_lon0,nav_h0,wgs84Ellipsoid);
    pos_es_ECEF(3) = depth;
end

== matlab function sim_all/EKF/SOS_flag_generator/MATLAB Function ==
  data: P_es input; SOS output; DVL input; AHRS input; gyro input; contatore input size=3 1; contatore output
%% Generazione flag di emergenza
% 1. Assenza di segnali dai sensori per un determinato tempo

function [SOS, contatore] = SOS_flag(P_es, DVL, AHRS, gyro, contatore)
    SOS=0;
 
    soglia_P = 10; %[m^2]
    if P_es(1,1)+P_es(2,2) > soglia_P || P_es(3,3) > soglia_P
        SOS=1;
    end
    
    if DVL == 1 
        contatore(1) = contatore(1) + 1;
    else
        contatore(1) = 0;
    end
    
    if AHRS == 1 
        contatore(2) = contatore(2) + 1;
    else
        contatore(2) = 0;
    end
    
    if gyro == 1 
        contatore(3) = contatore(3) + 1;
    else
        contatore(3) = 0;
    end
    
    if max(contatore) > 50 %50 equivale a 5 secondi
        SOS=1;
    end
    
    

end

== matlab function sim_all/Mission_supervisor_v3/Mission_Supervisor/Orientazione in profondità/MATLAB Function ==
  data: delta_current_or_prof output; delta_stato_or_prof output; Pos_d output size=3; Dpp_d output; Orp_d output; Pos_s input; Orp_s input; relativeDirection parameter; depth parameter; punto_iniz_patt input; error_flag input; soglia_orp parameter; soglia_SOS_pos parameter; SOS parameter; distanceFromWall parameter
function [delta_current_or_prof, delta_stato_or_prof, Pos_d, Dpp_d, Orp_d] = Orientazione_profondita(Pos_s, Orp_s, relativeDirection, depth, punto_iniz_patt, error_flag, soglia_orp, soglia_SOS_pos, SOS, distanceFromWall)

    disp("Orientazione in profondita");
    
    %% Unità di misura 
    
    % Pos_d, Pos_s, punto_iniz_patt, soglia_SOS_pos                        [deg, deg, m]
    % Orp_d, Orp_s, soglia_orp                                             [rad]
    % relativeDirection                                                    [deg]
    % Dpp_d, depth, distanceFromWall                                       [m]

    %% Inizializzazione variabili
    
    % Utilizzata per la permanenza nello stato corrente
    delta_stato_or_prof = 0;
    
    pronti = false;

    %% Preparazione dei riferimenti da fornire ai blocchi successivi
                
    % Posizione da mantenere
    Pos_d = [punto_iniz_patt(1); punto_iniz_patt(2); depth];
                                                                            %*****TEST******%
                                                                            %Pos_d = [43; 11; 0];
    
  
    % Orientazione da raggiungere
    Orp_d = deg2rad(relativeDirection);
    
    % Distanza dalla parete da mantenere
    Dpp_d = distanceFromWall;
    
    
    % Transizione di stato effettiva
    delta_current_or_prof = 104 - 103; 
    
    
    %% Verifiche
    
    % Verifica della corretta posizione
    if (abs(Pos_s(1) - Pos_d(1)) > soglia_SOS_pos(1) || ...
        abs(Pos_s(2) - Pos_d(2)) > soglia_SOS_pos(2) || ...
        abs(Pos_s(3) - Pos_d(3)) > soglia_SOS_pos(3))
    
        SOS = 1;
        disp("EMERGENZA:");
        
        if (abs(Pos_s(1) - Pos_d(1)) > soglia_SOS_pos(1))
            disp("Rilevato errore sulla posizione X");
        end
        if (abs(Pos_s(2) - Pos_d(2)) > soglia_SOS_pos(2))
            disp("Rilevato errore sulla posizione Y");
        end
        if (abs(Pos_s(3) - Pos_d(3)) > soglia_SOS_pos(3))
            disp("Rilevato errore sulla profondita Z");
        end
        
    end
    
    if error_flag == 1
        disp("EMERGENZA: errore segnalato dagli altri sottosistemi");
        SOS = 1;
    end
     
    % Si verifica di aver raggiunto l'orientazione desiderata
    if (SOS == 0 && ...
        abs(Orp_s - Orp_d) < soglia_orp)
    
        pronti = true;
    end
    
    %% Decisione dello stato successivo
    
    if pronti == true
        
        delta_stato_or_prof = 201 - 104; % Transizione eseguita correttamente
    end
    if SOS == 1
            
            delta_stato_or_prof = 301 - 104; % Transizione nello stato di emergenza
    end
    
    % Si rimane nello stato corrente
    

end

== matlab function sim_all/Mission_supervisor_v3/Mission_Supervisor/Frenata pattugliamento/MATLAB Function ==
  data: delta_current_fren_patt output; delta_stato_fren_patt output; contatore input; Pos_d output size=3; Dpp_d output; Dps_d output; Orp_d output; Pos_s input; Dpp_s input; Dps_s input; Orp_s input; distanceFromWall parameter; relativeDirection parameter; depth parameter; error_flag input; soglia_SOS_orp parameter; soglia_SOS_pos parameter; soglia_SOS_parete parameter; SOS parameter; soglia_parete parameter
function [delta_current_fren_patt, delta_stato_fren_patt, Pos_d, Dpp_d, Dps_d, Orp_d] = Frenata_pattugliamento(contatore, Pos_s, Dpp_s, Dps_s, Orp_s, distanceFromWall, relativeDirection, depth, error_flag, soglia_SOS_orp, soglia_SOS_pos, soglia_SOS_parete, SOS,soglia_parete)

    disp("Frenata (durante il pattugliamento)");
    
    %% Unità di misura 
    
    % Pos_d, Pos_s, soglia_SOS_pos                                                                 [deg, deg, m]
    % Orp_d, Orp_s, soglia_SOS_orp                                                                 [rad]
    % relativeDirection                                                                            [deg]
    % Dpp_d, Dps_d, Dpp_s, Dps_s, distanceFromWall, depth, soglia_SOS_parete, soglia_parete        [m]

    %% Inizializzazione variabili
   
    % Utilizzata per permanere nello stato corrente
    delta_stato_fren_patt = contatore;
    
    pronti = false;
    
    %% Preparazione dei riferimenti da fornire ai blocchi successivi
    
    % Profondità da mantenere
    Pos_d = [nan; nan; depth];
                                                                            %*****TEST******%
                                                                            %Pos_d = [nan; nan; 0];
    
    % Distanza dalla parete da mantenere
    Dpp_d = distanceFromWall;
    Dps_d = distanceFromWall;
    
    % Orientazione da mantenere
    Orp_d = deg2rad(relativeDirection);
    
    % Transizione di stato effettiva
    delta_current_fren_patt = 202 - 201 + contatore;  
    
    
    %% Verifiche
    
    % Verifica sulla corretta orientazione, profondità e distanza dalla parete pattugliata
    if (abs(Orp_s - Orp_d) > soglia_SOS_orp || ...
        abs(Dpp_s - Dpp_d) > soglia_SOS_parete || ...
        abs(Pos_s(3) - Pos_d(3)) > soglia_SOS_pos(3))
    
        SOS = 1;
        disp("EMERGENZA:");
        
        if (abs(Orp_s - Orp_d) > soglia_SOS_orp)
            disp("Rilevato errore sull'orientazione relativa");
        end
        
        if (abs(Dpp_s - Dpp_d) > soglia_SOS_parete)
            disp("Rilevato errore sulla distanza da parete");
        end
        
        if (abs(Pos_s(3) - Pos_d(3)) > soglia_SOS_pos(3))
            disp("Rilevato errore sulla profondita Z");
        end
        
    end
    
    if error_flag == 1
        disp("EMERGENZA: errore segnalato dagli altri sottosistemi");
        SOS = 1;
    end
     
                                                                            %*****TEST******%
                                                                            %test=0;
                                                                            %Serve per testare di rimanere 
                                                                            %in attesa in questo stato
                                                                            % if(contatore>2)
                                                                            %    test=100;
                                                                            % else
                                                                            %    test=0;
                                                                            % end

    % Si verifica di aver raggiunto la posizione desiderata in termini di 
    % distanza dalla parete successiva
    if (SOS == 0 && ...
        abs(Dps_s - Dps_d) < soglia_parete)
    
        pronti = true;
        
    end

    %% Decisione dello stato successivo
    
    if pronti == true
        
        delta_stato_fren_patt = 203 - 202 + contatore; % Transizione eseguita correttamente
    end
    if SOS == 1
            
            delta_stato_fren_patt = 301 - 202 + contatore; % Transizione nello stato di emergenza
    end
    % Si rimane nello stato corrente

end
